simulink model "Double_Pendulum_Calculations"  (R2022b)
settings: Solver=ode23t  StartTime=0.0  StopTime=50  MaxStep=0.01*1.6  RelTol=1e-3
libraries: simulink_extras x4
settings Model: Creator=lukac  LastModifiedBy=lukac
settings SolverCC: MaxConsecutiveZCs=1  MaxConsecutiveMinStep=100  ZeroCrossAlgorithm=Adaptive
settings DebuggingCC: IgnoredZcDiagnostic=none  UnconnectedInputMsg=warning  UnconnectedOutputMsg=warning  UnconnectedLineMsg=warning  SFMachineParentedDataDiag=warning
settings ModelReferenceCC: EnableRefExpFcnMdlSchedulingChecks=on
settings RTWCC: DLArmComputeVersion=19.05

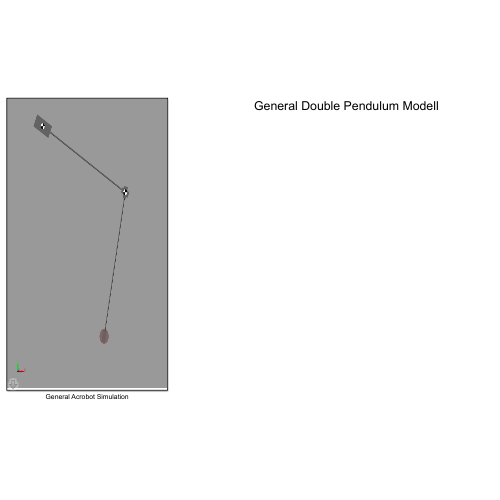
[thumbnail: Simulink's stored preview of the top-level diagram]
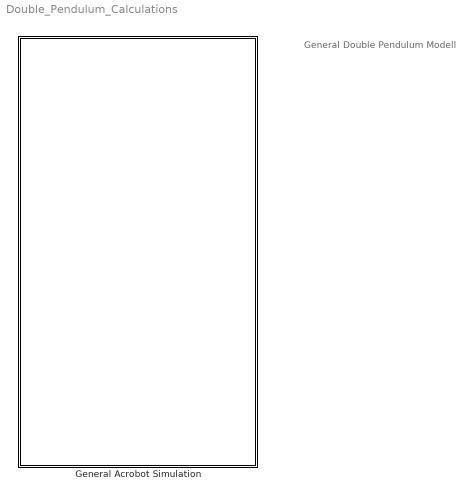
== system Double_Pendulum_Calculations ==
  note: General Double Pendulum Modell
  General Acrobot Simulation : Subsystem  mask{m1=1, m2=1, l1=0.6, l2=1, lc1=0.2, lc2=0.5, Q0=[pi+0.17 0.0 0.0 0.0]}
      mask prompts: m1 "Mass1 [kg]"; m2 "Mass2 [kg]"; l1 "Length1 [m]"; l2 "Length2 [m]"; lc1 "Length COM1 [m]"; lc2 "Length COM2 [m]"; Q0 "Initial state [q1 dq1 q2 dq2]  [rad]"
      mask Display: image('Acrobot_modell_subsys2.png'); % Use "Edit Image" on toolstrip to change.

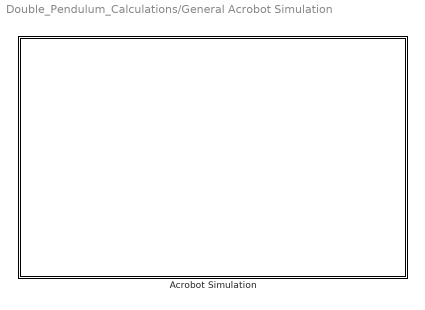
== system Double_Pendulum_Calculations/General Acrobot Simulation ==
  Acrobot Simulation : Subsystem

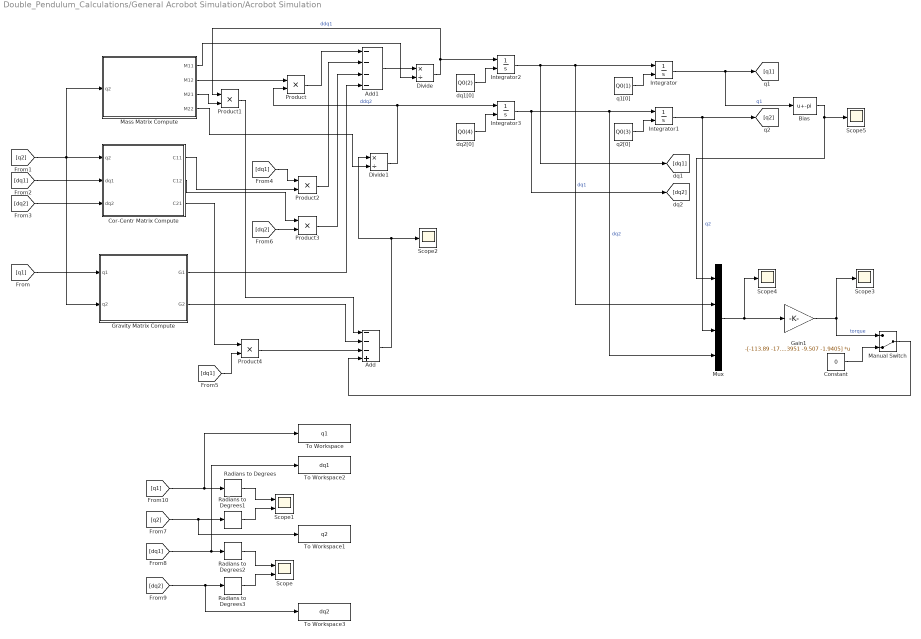
== system Double_Pendulum_Calculations/General Acrobot Simulation/Acrobot Simulation ==
  Add : Sum  Inputs=---+
  Add1 : Sum  Inputs=----
  Bias : Bias  Bias=-pi  SaturateOnIntegerOverflow=off
  Constant : Constant  Value=0
  Cor-Centr Matrix Compute : Subsystem
  Divide : Product  Inputs=*/
  Divide1 : Product  Inputs=*/
  Gain1 : Gain  Gain=-[-113.89 -17.3951 -9.507 -1.9405]  Multiplication=Matrix(K*u)
  Gravity Matrix Compute : Subsystem
  Integrator : Integrator  InitialConditionSource=external
  Integrator1 : Integrator  InitialConditionSource=external  InitialCondition=pi/6
  Integrator2 : Integrator  InitialConditionSource=external
  Integrator3 : Integrator  InitialConditionSource=external
  Manual Switch : ManualSwitch  CurrentSetting=0
  Mass Matrix Compute : Subsystem
  Mux : Mux
  Product{,1..4} (5 alike) : Product
  Radians to Degrees{,1..3} (4 alike) : simulink_extras/Transformations/Radians to Degrees
  Scope : Scope  NumInputPorts=2
  Scope1 : Scope  NumInputPorts=2
  Scope{2..5} (4 alike) : Scope
  To Workspace : ToWorkspace  VariableName=q1  SaveFormat=Timeseries  SampleTime=-1
  To Workspace1 : ToWorkspace  VariableName=q2  SaveFormat=Timeseries  SampleTime=-1
  To Workspace2 : ToWorkspace  VariableName=dq1  SaveFormat=Timeseries  SampleTime=-1
  To Workspace3 : ToWorkspace  VariableName=dq2  SaveFormat=Timeseries  SampleTime=-1
  dq1[0] : Constant  Value=Q0(2)
  dq2[0] : Constant  Value=Q0(4)
  q1[0] : Constant  Value=Q0(1)  VectorParams1D=off
  q2[0] : Constant  Value=Q0(3)
  wires:
  [dq2] -> To Workspace3/1, Radians to Degrees3/1
  Gravity Matrix Compute/2(G2) -> Add/2
  Integrator1/1 -> [q2], Mux/3  "q2"
  Product/1 -> Add1/1
  [dq2] -> Product3/2
  [dq1] -> Product4/2
  Gain1/1 -> Scope3/1, Manual Switch/1  "torque"
  Divide/1 -> Integrator2/1, Product1/1  "ddq1"
  [q2] -> Gravity Matrix Compute/2(q2), Cor-Centr Matrix Compute/1(q2), Mass Matrix Compute/1(q2)
  Add/1 -> Scope2/1, Divide1/1
  Cor-Centr Matrix Compute/1(C11) -> Product2/2
  Gravity Matrix Compute/1(G1) -> Add1/4
  q2[0]/1 -> Integrator1/2
  [dq1] -> To Workspace2/1, Radians to Degrees2/1
  q1[0]/1 -> Integrator/2
  dq2[0]/1 -> Integrator3/2
  [dq1] -> Product2/1
  [dq2] -> Cor-Centr Matrix Compute/3(dq2)
  Radians to Degrees/1 -> Scope1/1
  Mass Matrix Compute/2(M12) -> Product/1
  [dq1] -> Cor-Centr Matrix Compute/2(dq1)
  dq1[0]/1 -> Integrator2/2
  Integrator3/1 -> Mux/4, Integrator1/1, [dq2]  "dq2"
  Integrator2/1 -> Mux/2, Integrator/1, [dq1]  "dq1"
  Radians to Degrees1/1 -> Scope1/2
  Mass Matrix Compute/4(M22) -> Divide1/2
  [q1] -> Gravity Matrix Compute/1(q1)
  Divide1/1 -> Integrator3/1, Product/2  "ddq2"
  Product1/1 -> Add/1
  Mass Matrix Compute/1(M11) -> Divide/2
  Product3/1 -> Add1/3
  Add1/1 -> Divide/1
  Cor-Centr Matrix Compute/2(C12) -> Product3/1
  Cor-Centr Matrix Compute/3(C21) -> Product4/1
  Product2/1 -> Add1/2
  Mass Matrix Compute/3(M21) -> Product1/2
  Radians to Degrees3/1 -> Scope/2
  [q2] -> To Workspace1/1, Radians to Degrees1/1
  [q1] -> To Workspace/1, Radians to Degrees/1
  Radians to Degrees2/1 -> Scope/1
  Product4/1 -> Add/3
  Bias/1 -> Mux/1, Scope5/1
  Integrator/1 -> Bias/1, [q1]  "q1"
  Mux/1 -> Gain1/1, Scope4/1
  Manual Switch/1 -> Add/4
  Constant/1 -> Manual Switch/2

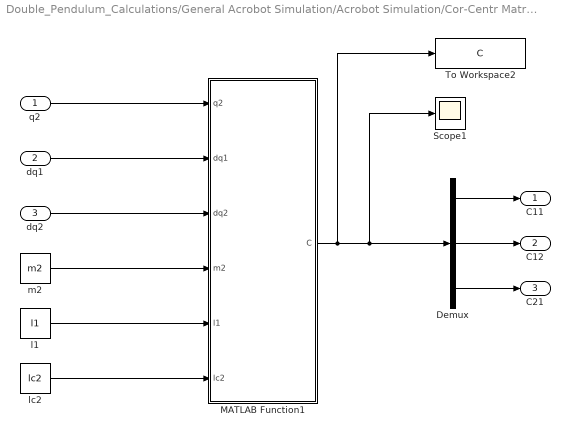
== system Double_Pendulum_Calculations/General Acrobot Simulation/Acrobot Simulation/Cor-Centr Matrix Compute ==
  q2 : Inport
  dq1 : Inport  Port=2
  dq2 : Inport  Port=3
  Demux : Demux  Outputs=3
  MATLAB Function1 : MATLAB Function  TreatAsAtomicUnit=on
  Scope1 : Scope
  To Workspace2 : ToWorkspace  VariableName=C  SaveFormat=Timeseries  SampleTime=-1
  l1 : Constant  Value=l1
  lc2 : Constant  Value=lc2
  m2 : Constant  Value=m2
  C11 : Outport
  C12 : Outport  Port=2
  C21 : Outport  Port=3
  wires:
  Demux/1 -> C11/1
  Demux/2 -> C12/1
  Demux/3 -> C21/1
  MATLAB Function1/1(C) -> To Workspace2/1, Scope1/1, Demux/1
  q2/1 -> MATLAB Function1/1(q2)
  dq1/1 -> MATLAB Function1/2(dq1)
  dq2/1 -> MATLAB Function1/3(dq2)
  m2/1 -> MATLAB Function1/4(m2)
  l1/1 -> MATLAB Function1/5(l1)
  lc2/1 -> MATLAB Function1/6(lc2)

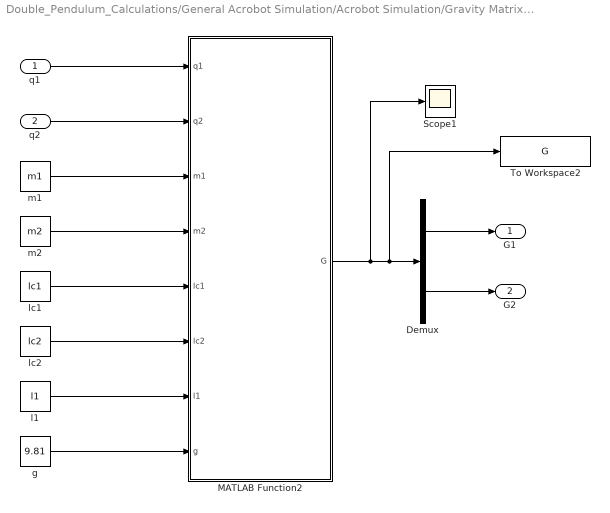
== system Double_Pendulum_Calculations/General Acrobot Simulation/Acrobot Simulation/Gravity Matrix Compute ==
  q1 : Inport
  q2 : Inport  Port=2
  Demux : Demux  Outputs=2
  MATLAB Function2 : MATLAB Function  TreatAsAtomicUnit=on
  Scope1 : Scope
  To Workspace2 : ToWorkspace  VariableName=G  SaveFormat=Timeseries  SampleTime=-1
  g : Constant  Value=9.81
  l1 : Constant  Value=l1
  lc1 : Constant  Value=lc1
  lc2 : Constant  Value=lc2
  m1 : Constant  Value=m1
  m2 : Constant  Value=m2
  G1 : Outport
  G2 : Outport  Port=2
  wires:
  Demux/1 -> G1/1
  Demux/2 -> G2/1
  MATLAB Function2/1(G) -> Scope1/1, To Workspace2/1, Demux/1
  q1/1 -> MATLAB Function2/1(q1)
  q2/1 -> MATLAB Function2/2(q2)
  g/1 -> MATLAB Function2/8(g)
  m1/1 -> MATLAB Function2/3(m1)
  m2/1 -> MATLAB Function2/4(m2)
  lc1/1 -> MATLAB Function2/5(lc1)
  lc2/1 -> MATLAB Function2/6(lc2)
  l1/1 -> MATLAB Function2/7(l1)

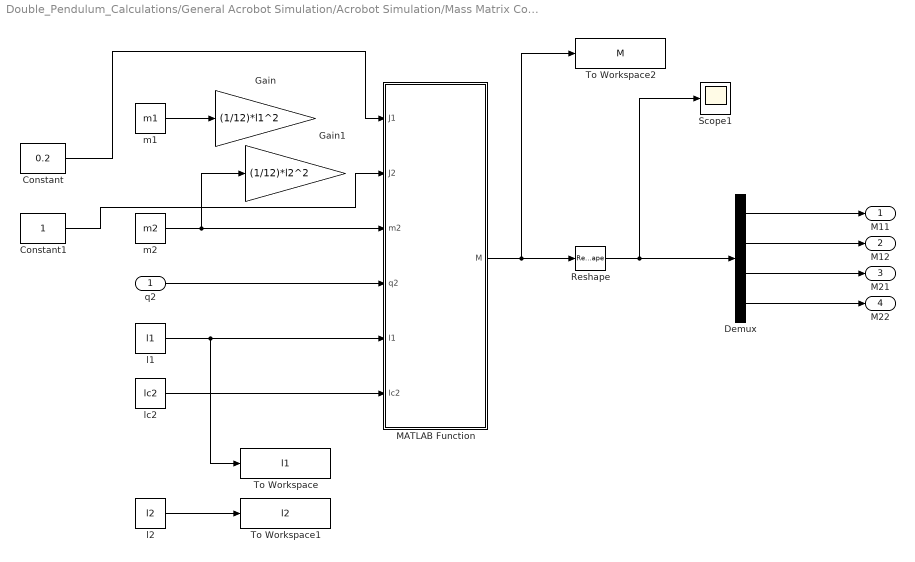
== system Double_Pendulum_Calculations/General Acrobot Simulation/Acrobot Simulation/Mass Matrix Compute ==
  q2 : Inport
  Constant : Constant  Value=0.2
  Constant1 : Constant
  Demux : Demux
  Gain : Gain  Gain=(1/12)*l1^2
  Gain1 : Gain  Gain=(1/12)*l2^2
  MATLAB Function : MATLAB Function  TreatAsAtomicUnit=on
  Reshape : Reshape
  Scope1 : Scope
  To Workspace : ToWorkspace  VariableName=l1  SaveFormat=Timeseries  SampleTime=-1
  To Workspace1 : ToWorkspace  VariableName=l2  SaveFormat=Timeseries  SampleTime=-1
  To Workspace2 : ToWorkspace  VariableName=M  SaveFormat=Timeseries  SampleTime=-1
  l1 : Constant  Value=l1
  l2 : Constant  Value=l2
  lc2 : Constant  Value=lc2
  m1 : Constant  Value=m1
  m2 : Constant  Value=m2
  M11 : Outport
  M12 : Outport  Port=2
  M21 : Outport  Port=3
  M22 : Outport  Port=4
  wires:
  MATLAB Function/1(M) -> To Workspace2/1, Reshape/1
  Reshape/1 -> Scope1/1, Demux/1
  Demux/1 -> M11/1
  Demux/2 -> M12/1
  Demux/3 -> M21/1
  Demux/4 -> M22/1
  q2/1 -> MATLAB Function/4(q2)
  m2/1 -> Gain1/1, MATLAB Function/3(m2)
  l1/1 -> To Workspace/1, MATLAB Function/5(l1)
  lc2/1 -> MATLAB Function/6(lc2)
  m1/1 -> Gain/1
  l2/1 -> To Workspace1/1
  Constant/1 -> MATLAB Function/1(J1)
  Constant1/1 -> MATLAB Function/2(J2)

== matlab function Double_Pendulum_Calculations/General Acrobot Simulation/Acrobot Simulation/Cor-Centr Matrix Compute/MATLAB Function1 ==
  data: q2 input; dq1 input; dq2 input; C output; m2 input; l1 input; lc2 input
function C = C_matrix(q2,dq1,dq2,m2,l1,lc2)

C1 = -2*m2*l1*lc2*sin(q2)*dq2;
C2 = -m2*l1*lc2*sin(q2)*dq2;
C3 = m2*l1*lc2*sin(q2)*dq1;
%C4 = 0;

C = [C1;C2;C3];

end

== matlab function Double_Pendulum_Calculations/General Acrobot Simulation/Acrobot Simulation/Mass Matrix Compute/MATLAB Function ==
  data: J1 input; J2 input; m2 input; M output; q2 input; l1 input; lc2 input
function M = Mass_matrix(J1,J2,m2,q2,l1,lc2)

%M11 = alfa1 + alfa2 + 2*alfa3*cos(q2);
%M12 = alfa2 + alfa3*cos(q2);
%M21 = M12;
%M22 = alfa2;

M11 = J1+J2+m2*l1^2+2*m2*l1*lc2*cos(q2);
M12 = J2 + m2*l1*lc2*cos(q2);
M21 = M12;
M22 = J2;

M = [M11 M12; M21 M22];

end

== matlab function Double_Pendulum_Calculations/General Acrobot Simulation/Acrobot Simulation/Gravity Matrix Compute/MATLAB Function2 ==
  data: G output; q1 input; q2 input; m1 input; m2 input; lc1 input; lc2 input; l1 input; g input
function G = Gravity_matrix(q1,q2,m1,m2,lc1,lc2,l1,g)

G1 = m1*g*lc1*sin(q1) + m2*g*(l1*sin(q1)+lc2*sin(q1+q2));
G2 = m2*g*lc2*sin(q1+q2);

G = [G1;G2];

end
